simulink model "sldemo_mdlref_depgraph"  (R2019b)
settings: Solver=ode3  StartTime=0.0  StopTime=2*24*60*60  FixedStep=60  RelTol=1e-3  AbsTol=1e-6
settings Model: ModifiedByFormat=The MathWorks Inc.  ExtModeTrigMode=oneshot  ExtModeArmWhenConnect=off  ExtModeAutoUpdateStatusClock=off  Creator=The MathWorks, Inc.  LastModifiedBy=The MathWorks Inc.
settings SolverCC: AutoScaleAbsTol=off
settings DataIOCC: ExternalInput=[]  InitialState=[]  SaveFormat=Array  SaveOutput=off  SaveTime=off  ReturnWorkspaceOutputs=off
settings OptimizationCC: BlockReduction=off  BooleanDataType=off  DefaultParameterBehavior=Inlined  InlineInvariantSignals=on  ExpressionDepthLimit=2147483647  InitFltsAndDblsToZero=on  LifeSpan=inf
settings DebuggingCC: SaveWithParameterizedLinksMsg=none  CheckExecutionContextPreStartOutputMsg=on  CheckExecutionContextRuntimeOutputMsg=on  MultiTaskDSMMsg=warning  MultiTaskCondExecSysMsg=none  SigSpecEnsureSampleTimeMsg=none  IntegerOverflowMsg=none  FcnCallInpInsideContextMsg=warning  StateNameClashWarn=warning  SFUnexpectedBacktrackingDiag=warning  SFNoUnconditionalDefaultTransitionDiag=warning  SFExecutionAtInitializationDiag=none  IntegerSaturationMsg=none  ArithmeticOperatorsInVariantConditions=warning
settings HardwareCC: ProdBitPerPointer=32  ProdBitPerSizeT=32  ProdBitPerPtrDiffT=32  ProdLargestAtomicFloat=None  ProdIntDivRoundTo=Undefined  ProdEndianess=Unspecified  ProdWordSize=32  ProdHWDeviceType=32-bit Generic
settings ModelReferenceCC: UpdateModelReferenceTargets=IfOutOfDate  PropagateSignalLabelsOutOfModel=off
settings SFSimCC: SimUseLocalCustomCode=off  CustomCodeUndefinedFunction=UseInterfaceOnly
settings RTWCC: RTWUseLocalCustomCode=off
settings CodeAppCC: MaxIdLength=100  StateflowObjectComments=on
settings GRTTargetCC: TargetFcnLib=ansi_tfl_tmw.mat  TargetLangStandard=C89/C90 (ANSI)  GeneratePreprocessorConditionals=Disable all  CombineOutputUpdateFcns=off  GRTInterface=on
settings ConfigComp: CovMetricSettings=dw  CovHtmlReporting=on  CovSaveCumulativeToWorkspaceVar=on  CovSaveSingleToWorkspaceVar=on  CovExternalEMLEnable=off  CovSFcnEnable=off

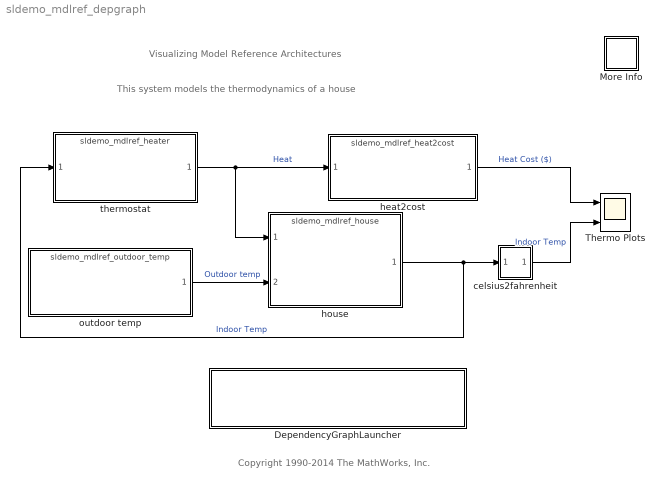
== system sldemo_mdlref_depgraph ==
  note: Visualizing Model Reference Architectures
  note: This system models the thermodynamics of a house
  note: Copyright 1990-2014 The MathWorks, Inc.
  DependencyGraphLauncher : Subsystem
      settings: OpenFcn=|
      | mdlName= get_param(bdroot(gcbh),'name');
      | view_mdlrefs(mdlName);
      mask Display: disp('Double click here to view \n Model Reference dependency graph');
  More Info : Subsystem
      settings: OpenFcn=showdemo(bdroot(gcb))
      mask Display: disp('?')
  Thermo Plots : Scope  NumInputPorts=2
  celsius2fahrenheit : Subsystem  mask(CelsiusToFahrenheit){}
      mask help:
      | Conversion from degrees Celsius to degrees Fahrenheit.
      |
      | F=9/5*C+32
      mask Help: This block converts from degrees Celsius to degrees Fahrenheit.
      mask Display: disp('C2F')
  heat2cost : ModelReference  ModelNameDialog=sldemo_mdlref_heat2cost  ModelReferenceVersion=1.17
  house : ModelReference  ModelNameDialog=sldemo_mdlref_house  ModelReferenceVersion=1.20
  outdoor temp : ModelReference  ModelNameDialog=sldemo_mdlref_outdoor_temp  ModelReferenceVersion=1.23
  thermostat : ModelReference  ModelNameDialog=sldemo_mdlref_heater  SimulationMode=Normal  ModelReferenceVersion=1.31
  wires:
  thermostat/1 -> house/1, heat2cost/1  "Heat"
  house/1 -> celsius2fahrenheit/1(Celsius in), thermostat/1  "Indoor Temp"
  outdoor temp/1 -> house/2  "Outdoor temp"
  heat2cost/1 -> Thermo Plots/1  "Heat Cost ($)"
  celsius2fahrenheit/1(Fahrenheit out) -> Thermo Plots/2  "Indoor Temp"

== system sldemo_mdlref_depgraph/DependencyGraphLauncher ==

== system sldemo_mdlref_depgraph/More Info ==
  note: Bus Block Demonstration
  note: This demonstration shows how signals may be grouped and ungrouped while
      | retaining their names.  In this demonstration, 5 signals are created and labelled
      | appropriately.  These signals are then mux'd together to create a bus of signals.
      | This bus of signals is then fed into the Bus Selector block.  Inside of the Bus
      | Selector block, the Pulse and Chirp signals are chosen to be output from the
      | original signal bus.
      |
      | It is possible to place a nest signal buses and then still retrieve the original signal
      | with its label.

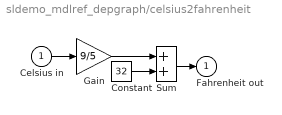
== system sldemo_mdlref_depgraph/celsius2fahrenheit ==
  Celsius in : Inport
  Constant : Constant  Value=32  OutDataTypeStr=Inherit: Inherit via back propagation
  Gain : Gain  Gain=9/5  SaturateOnIntegerOverflow=on  OutDataTypeStr=Inherit: Same as input  ParamDataTypeStr=Inherit: Same as input
  Sum : Sum  SaturateOnIntegerOverflow=on  InputSameDT=on  OutDataTypeStr=Inherit: Same as first input
  Fahrenheit out : Outport  InitialOutput=0  VectorParamsAs1DForOutWhenUnconnected=off
  wires:
  Celsius in/1 -> Gain/1
  Gain/1 -> Sum/1
  Sum/1 -> Fahrenheit out/1
  Constant/1 -> Sum/2
